simulink model "eps3"  (Simulink 8.3)
settings: Solver=ode3  SolverMode=SingleTasking  StartTime=0.0  StopTime=20  FixedStep=0.001  MaxStep=0.1  MinStep=0.01  RelTol=0.01
undefined symbols (not defined in the file or in its folder): Bc, Bm, G, Jc, Jm, Kc, Ke, Kt, L, R
libraries: fuzblock x2, Solver_SF x1
settings Model: Creator=xl  LastModifiedBy=汪天祥  CovMetricSettings=dwe  CovHtmlReporting=off  covSaveCumulativeToWorkspaceVar=off  CovSaveSingleToWorkspaceVar=off  CovExternalEMLEnable=on  CovSFcnEnable=on
settings SolverCC: InitialStep=0.01  ZeroCrossControl=EnableAll
settings DataIOCC: LimitDataPoints=off  SaveFormat=StructureWithTime  SignalLoggingSaveFormat=Dataset
settings DebuggingCC: UnderspecifiedInitializationDetection=Simplified  MergeDetectMultiDrivingBlocksExec=error  MaxConsecutiveZCsMsg=none  SolverPrmCheckMsg=none  FrameProcessingCompatibilityMsg=error  StateNameClashWarn=none  SFUnexpectedBacktrackingDiag=error  SFNoUnconditionalDefaultTransitionDiag=error
settings HardwareCC: ProdBitPerPointer=64  ProdLargestAtomicFloat=Float  ProdIntDivRoundTo=Zero  ProdEndianess=LittleEndian  ProdHWDeviceType=Specified
settings ModelReferenceCC: PropagateSignalLabelsOutOfModel=on
settings GRTTargetCC: TargetLangStandard=C99 (ISO)  GeneratePreprocessorConditionals=Use local settings  CombineOutputUpdateFcns=on  GRTInterface=off

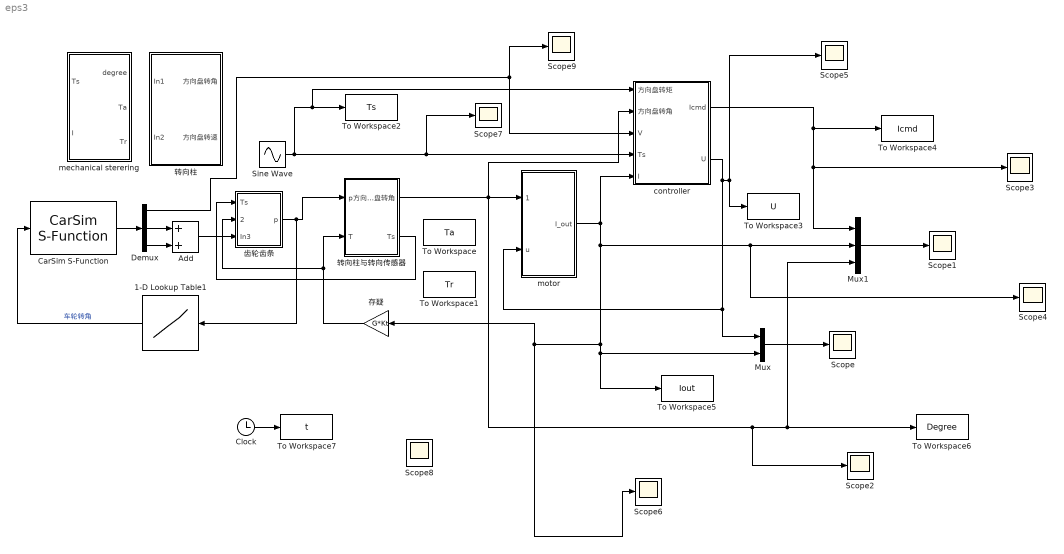
== system eps3 ==
  1-D Lookup Table1 : Lookup_n-D  NumberOfTableDimensions=1  BreakpointsForDimension1=[0 5 10 15 20 25 30 35 40 45 50 55 60 65 70 75 80]  Table=[2 4 6 8 10 12 14 16 18 20 22 24 27 29 31 33 36]  InternalRulePriority=Speed  RndMeth=Simplest  InputSameDT=on
  Add : Sum
  CarSim S-Function : Solver_SF/CarSim S-Function  Priority=1  VehicleCode=i_i  SIMFILE=simfile.sim
  Clock : Clock
  Demux : Demux  Outputs=3
  Mux : Mux  Inputs=2
  Mux1 : Mux  Inputs=3
  Scope{,1..9} (10 alike) : Scope
      Scope settings: YMin=-15.00000  YMax=15.00000
      Scope1 settings: YMin=-11.70772  YMax=11.82102
      Scope2 settings: YMin=-0.29342  YMax=0.29316
      Scope3 settings: YMin=-11.66423  YMax=11.66428  SaveName=ScopeData2  MaxDataPoints=10000
      Scope4 settings: YMin=-10  YMax=10  SaveName=ScopeData3
      Scope5 settings: YMin=-12.5  YMax=12.5  SaveName=ScopeData4
      Scope6 settings: YMin=-2.37496  YMax=2.36992  SaveName=ScopeData5
      Scope7 settings: YMin=-4.99999  YMax=5.00000  SaveName=ScopeData6
      Scope8 settings: YMin=-6.30329  YMax=6.29326  SaveName=ScopeData14
      Scope9 settings: YMin=-8.29353  YMax=8.28087  SaveName=ScopeData15
  Sine Wave : Sin  Amplitude=4  Frequency=1.333  SampleTime=0
  To Workspace : ToWorkspace  VariableName=Ta  SaveFormat=Timeseries  SampleTime=-1
  To Workspace1 : ToWorkspace  VariableName=Tr  SaveFormat=Timeseries  SampleTime=-1
  To Workspace2 : ToWorkspace  VariableName=Ts  SaveFormat=Timeseries  SampleTime=-1
  To Workspace3 : ToWorkspace  VariableName=U  SaveFormat=Timeseries  SampleTime=-1
  To Workspace4 : ToWorkspace  VariableName=Icmd  SaveFormat=Timeseries  SampleTime=-1
  To Workspace5 : ToWorkspace  VariableName=Iout  SaveFormat=Timeseries  SampleTime=-1
  To Workspace6 : ToWorkspace  VariableName=Degree  SaveFormat=Timeseries  SampleTime=-1
  To Workspace7 : ToWorkspace  VariableName=t  SaveFormat=Timeseries  SampleTime=-1
  "controller  " : Subsystem
  "mechanical sterering " : Subsystem
  "motor " : Subsystem
  存疑 : Gain  Gain=G*Kt
  转向柱 : Subsystem
  转向柱与转向传感器 : Subsystem
  齿轮齿条 : Subsystem
  wires:
  Sine Wave/1 -> "controller  "/1(方向盘转矩), To Workspace2/1, Scope7/1, "controller  "/4(Ts)
  "controller  "/2(U) -> "motor "/2(u), Mux/1, Scope5/1, To Workspace3/1
  "controller  "/1(Icmd) -> Scope3/1, Mux1/1, To Workspace4/1
  "motor "/1(I_out) -> Mux/2, To Workspace5/1, Scope6/1, 存疑/1, Scope4/1, Mux1/2, "controller  "/5(I)
  Mux/1 -> Scope/1
  Mux1/1 -> Scope1/1
  Clock/1 -> To Workspace7/1
  转向柱与转向传感器/1(方向盘转角) -> "controller  "/2(方向盘转角), "motor "/1("degree "), Scope2/1, To Workspace6/1, Mux1/3
  存疑/1 -> 转向柱与转向传感器/2(T), 齿轮齿条/2(电机转矩)
  齿轮齿条/1(p) -> 1-D Lookup Table1/1, 转向柱与转向传感器/1(p)
  转向柱与转向传感器/2(Ts) -> 齿轮齿条/1(Ts)
  Demux/1 -> Scope9/1, "controller  "/3(V)
  CarSim S-Function/1 -> Demux/1
  Demux/2 -> Add/1
  Demux/3 -> Add/2
  Add/1 -> 齿轮齿条/3(In3)
  1-D Lookup Table1/1 -> CarSim S-Function/1  "车轮转角"

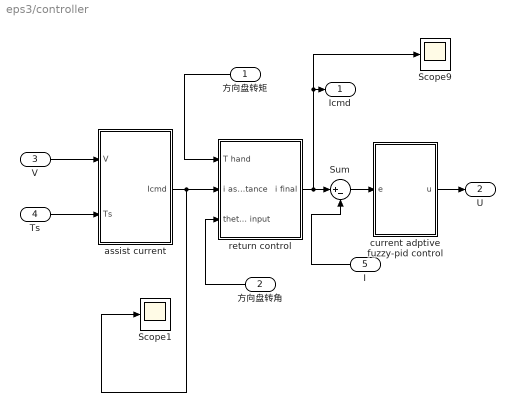
== system eps3/controller   ==
  方向盘转矩 : Inport
  方向盘转角 : Inport  Port=2
  V : Inport  Port=3
  Ts : Inport  Port=4
  I : Inport  Port=5
  Scope1 : Scope
      settings: YMin=-8.29353  YMax=8.28087  SaveName=ScopeData21
  Scope9 : Scope
      settings: YMin=-8.29353  YMax=8.28087  SaveName=ScopeData20
  Sum : Sum  Inputs=|+-
  "assist current " : Subsystem
  "current adptive fuzzy-pid control " : Subsystem
  "return control " : Subsystem
  Icmd : Outport
  U : Outport  Port=2
  wires:
  I/1 -> Sum/2
  "current adptive fuzzy-pid control "/1(u) -> U/1
  Sum/1 -> "current adptive fuzzy-pid control "/1("e ")
  V/1 -> "assist current "/1(V)
  Ts/1 -> "assist current "/2(Ts)
  方向盘转矩/1 -> "return control "/1("T hand ")
  方向盘转角/1 -> "return control "/3("theta input ")
  "assist current "/1(Icmd) -> Scope1/1, "return control "/2(i assitance)
  "return control "/1(i final) -> Scope9/1, Icmd/1, Sum/1

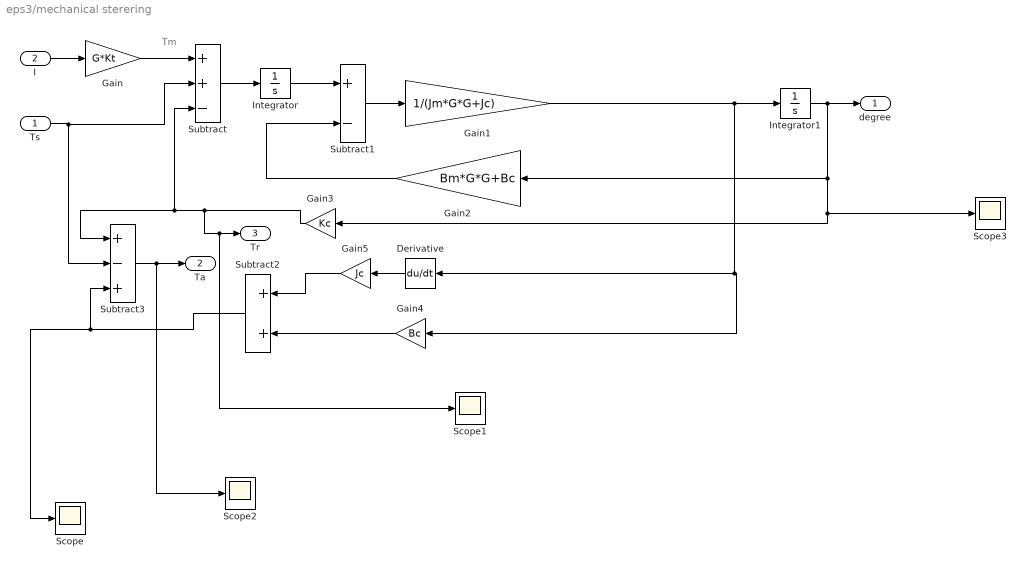
== system eps3/mechanical sterering  ==
  note: Tm
  Ts : Inport
  I : Inport  Port=2
  Derivative : Derivative
  Gain : Gain  Gain=G*Kt
  Gain1 : Gain  Gain=1/(Jm*G*G+Jc)
  Gain2 : Gain  Gain=Bm*G*G+Bc
  Gain3 : Gain  Gain=Kc
  Gain4 : Gain  Gain=Bc
  Gain5 : Gain  Gain=Jc
  Integrator : Integrator
  Integrator1 : Integrator
  Scope{,1..3} (4 alike) : Scope
      Scope settings: YMin=-0.17619  YMax=0.17432  SaveName=ScopeData16
      Scope1 settings: YMin=-13.24776  YMax=13.23609  SaveName=ScopeData17
      Scope2 settings: YMin=-8.29353  YMax=8.28087  SaveName=ScopeData18
      Scope3 settings: YMin=-0.13961  YMax=0.13939  SaveName=ScopeData19
  Subtract : Sum  Inputs=++-
  Subtract1 : Sum  Inputs=+-
  Subtract2 : Sum
  Subtract3 : Sum  Inputs=+-+
  "degree " : Outport
  Ta : Outport  Port=2
  Tr : Outport  Port=3
  wires:
  Subtract2/1 -> Scope/1, Subtract3/3
  Gain5/1 -> Subtract2/1
  Gain4/1 -> Subtract2/2
  Derivative/1 -> Gain5/1
  Gain2/1 -> Subtract1/2
  Integrator1/1 -> "degree "/1, Scope3/1, Gain3/1, Gain2/1
  Ts/1 -> Subtract/2, Subtract3/2
  Subtract3/1 -> Scope2/1, Ta/1
  Gain3/1 -> Scope1/1, Tr/1, Subtract3/1, Subtract/3
  Gain/1 -> Subtract/1
  Integrator/1 -> Subtract1/1
  Gain1/1 -> Derivative/1, Gain4/1, Integrator1/1
  I/1 -> Gain/1
  Subtract/1 -> Integrator/1
  Subtract1/1 -> Gain1/1

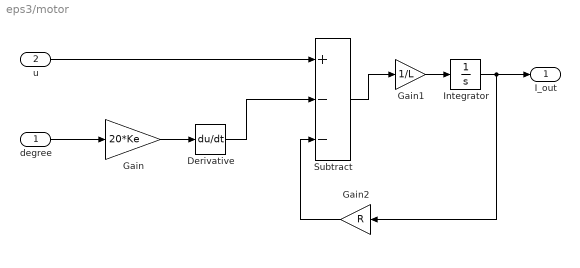
== system eps3/motor  ==
  "degree " : Inport
  u : Inport  Port=2
  Derivative : Derivative
  Gain : Gain  Gain=20*Ke
  Gain1 : Gain  Gain=1/L
  Gain2 : Gain  Gain=R
  Integrator : Integrator
  Subtract : Sum  Inputs=+--
  I_out : Outport
  wires:
  u/1 -> Subtract/1
  "degree "/1 -> Gain/1
  Derivative/1 -> Subtract/2
  Gain/1 -> Derivative/1
  Subtract/1 -> Gain1/1
  Gain2/1 -> Subtract/3
  Integrator/1 -> I_out/1, Gain2/1
  Gain1/1 -> Integrator/1

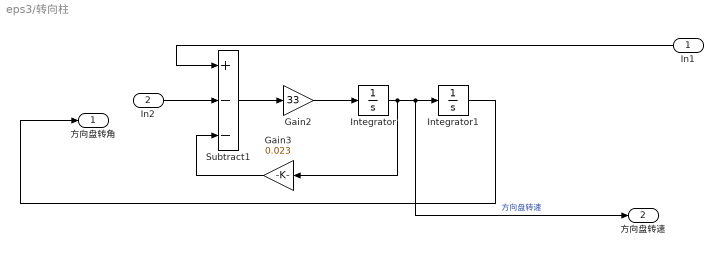
== system eps3/转向柱 ==
  In1 : Inport
  In2 : Inport  Port=2
  Gain2 : Gain  Gain=33
  Gain3 : Gain  Gain=0.023
  Integrator : Integrator
  Integrator1 : Integrator
  Subtract1 : Sum  Inputs=+--
  方向盘转角 : Outport
  方向盘转速 : Outport  Port=2
  wires:
  In2/1 -> Subtract1/2
  In1/1 -> Subtract1/1
  Integrator/1 -> Gain3/1, 方向盘转速/1, Integrator1/1  "方向盘转速"
  Integrator1/1 -> 方向盘转角/1
  Subtract1/1 -> Gain2/1
  Gain3/1 -> Subtract1/3
  Gain2/1 -> Integrator/1

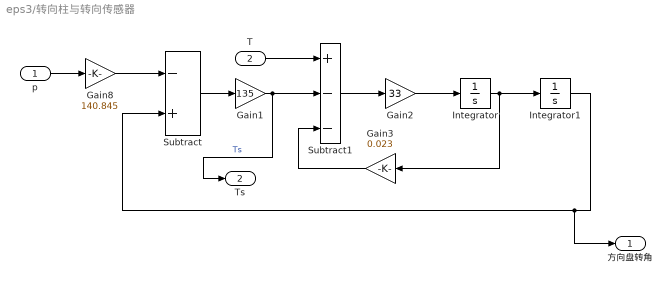
== system eps3/转向柱与转向传感器 ==
  p : Inport
  T : Inport  Port=2
  Gain1 : Gain  Gain=135
  Gain2 : Gain  Gain=33
  Gain3 : Gain  Gain=0.023
  Gain8 : Gain  Gain=140.845
  Integrator : Integrator
  Integrator1 : Integrator
  Subtract : Sum  Inputs=-+
  Subtract1 : Sum  Inputs=+--
  方向盘转角 : Outport
  Ts : Outport  Port=2
  wires:
  p/1 -> Gain8/1
  Gain1/1 -> Ts/1, Subtract1/2  "Ts"
  Gain2/1 -> Integrator/1
  Subtract/1 -> Gain1/1
  Subtract1/1 -> Gain2/1
  Integrator/1 -> Gain3/1, Integrator1/1
  T/1 -> Subtract1/1
  Integrator1/1 -> 方向盘转角/1, Subtract/2
  Gain3/1 -> Subtract1/3
  Gain8/1 -> Subtract/1

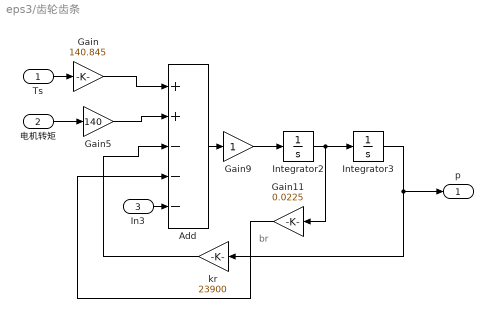
== system eps3/齿轮齿条 ==
  note: br
  Ts : Inport
  电机转矩 : Inport  Port=2
  In3 : Inport  Port=3
  Add : Sum  Inputs=++---
  Gain : Gain  Gain=140.845
  Gain11 : Gain  Gain=0.0225
  Gain5 : Gain  Gain=140
  Gain9 : Gain
  Integrator2 : Integrator
  Integrator3 : Integrator
  kr : Gain  Gain=23900
  p : Outport
  wires:
  Ts/1 -> Gain/1
  Add/1 -> Gain9/1
  Gain/1 -> Add/1
  kr/1 -> Add/3
  Gain5/1 -> Add/2
  Integrator2/1 -> Gain11/1, Integrator3/1
  Integrator3/1 -> p/1, kr/1
  Gain9/1 -> Integrator2/1
  Gain11/1 -> Add/4
  电机转矩/1 -> Gain5/1
  In3/1 -> Add/5

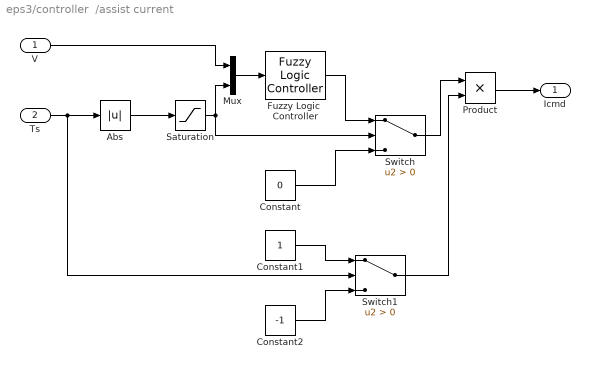
== system eps3/controller  /assist current  ==
  V : Inport
  Ts : Inport  Port=2
  Abs : Abs
  Constant : Constant  Value=0
  Constant1 : Constant
  Constant2 : Constant  Value=-1
  Fuzzy Logic  Controller : fuzblock/Fuzzy Logic  Controller  fis=assistcurrent
  Mux : Mux  Inputs=2
  Product : Product
  Saturation : Saturate  UpperLimit=80  LowerLimit=0
  Switch : Switch  Criteria=u2 > Threshold
  Switch1 : Switch  Criteria=u2 > Threshold
  Icmd : Outport
  wires:
  V/1 -> Mux/1
  Switch/1 -> Product/1
  Constant1/1 -> Switch1/1
  Switch1/1 -> Product/2
  Constant2/1 -> Switch1/3
  Mux/1 -> Fuzzy Logic  Controller/1
  Ts/1 -> Switch1/2, Abs/1
  Abs/1 -> Saturation/1
  Product/1 -> Icmd/1
  Saturation/1 -> Switch/2, Mux/2
  Constant/1 -> Switch/3
  Fuzzy Logic  Controller/1 -> Switch/1

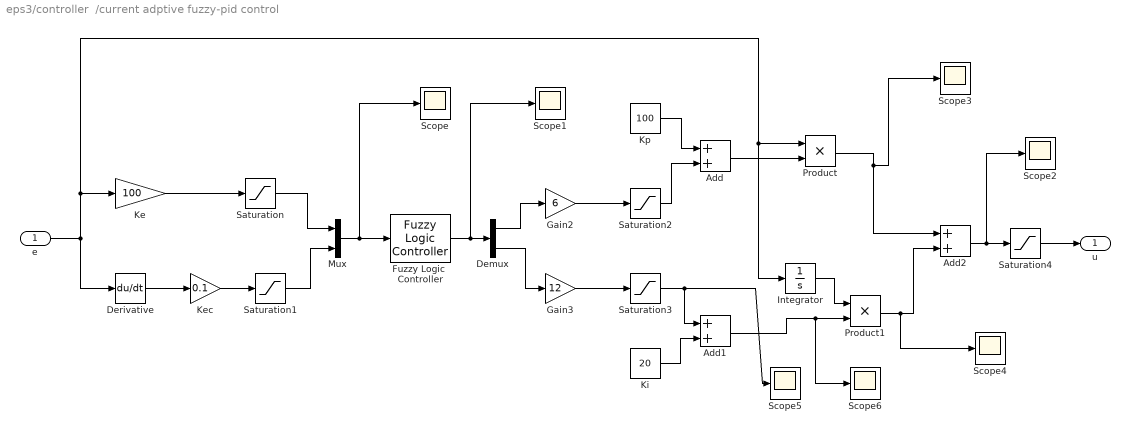
== system eps3/controller  /current adptive fuzzy-pid control  ==
  "e " : Inport
  Add : Sum
  Add1 : Sum
  Add2 : Sum
  Demux : Demux  Outputs=2
  Derivative : Derivative
  Fuzzy Logic  Controller : fuzblock/Fuzzy Logic  Controller  fis=adptivefuzzypidcontrol
  Gain2 : Gain  Gain=6
  Gain3 : Gain  Gain=12
  Integrator : Integrator
  Ke : Gain  Gain=100
  Kec : Gain  Gain=0.1
  Ki : Constant  Value=20
  Kp : Constant  Value=100
  Mux : Mux  Inputs=2
  Product : Product
  Product1 : Product
  Saturation{,1..3} (4 alike) : Saturate  UpperLimit=6  LowerLimit=-6
  Saturation4 : Saturate  UpperLimit=12  LowerLimit=-12
  Scope{,1..6} (7 alike) : Scope
      Scope settings: YMin=-7.5  YMax=7.5  SaveName=ScopeData7
      Scope1 settings: YMin=-6.71538  YMax=6.71538  SaveName=ScopeData8
      Scope2 settings: YMin=-80.22694  YMax=672.92649  SaveName=ScopeData9
      Scope3 settings: YMin=-80.64056  YMax=672.97051  SaveName=ScopeData10
      Scope4 settings: YMin=-80.64056  YMax=672.97051  SaveName=ScopeData11
      Scope5 settings: YMin=-80.64056  YMax=672.97051  SaveName=ScopeData12
      Scope6 settings: YMin=2.5  YMax=17.5  SaveName=ScopeData13
  u : Outport
  wires:
  Kec/1 -> Saturation1/1
  Derivative/1 -> Kec/1
  Gain3/1 -> Saturation3/1
  Ki/1 -> Add1/2
  Saturation4/1 -> u/1
  "e "/1 -> Derivative/1, Product/1, Integrator/1, Ke/1
  Mux/1 -> Scope/1, Fuzzy Logic  Controller/1
  Saturation3/1 -> Scope5/1, Add1/1
  Add/1 -> Product/2
  Fuzzy Logic  Controller/1 -> Scope1/1, Demux/1
  Demux/2 -> Gain3/1
  Product/1 -> Scope3/1, Add2/1
  Product1/1 -> Scope4/1, Add2/2
  Add2/1 -> Scope2/1, Saturation4/1
  Saturation/1 -> Mux/1
  Saturation1/1 -> Mux/2
  Integrator/1 -> Product1/1
  Add1/1 -> Scope6/1, Product1/2
  Gain2/1 -> Saturation2/1
  Demux/1 -> Gain2/1
  Saturation2/1 -> Add/2
  Kp/1 -> Add/1
  Ke/1 -> Saturation/1

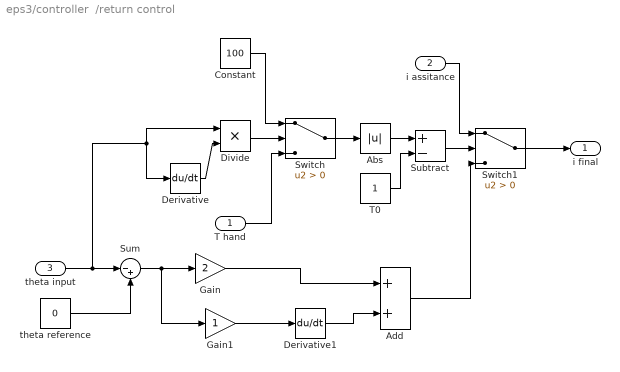
== system eps3/controller  /return control  ==
  "T hand " : Inport
  i assitance : Inport  Port=2
  "theta input " : Inport  Port=3
  Abs : Abs
  Add : Sum
  Constant : Constant  Value=100
  Derivative : Derivative
  Derivative1 : Derivative
  Divide : Product  Inputs=**
  Gain : Gain  Gain=2
  Gain1 : Gain
  Subtract : Sum  Inputs=+-
  Sum : Sum  Inputs=|-+
  Switch : Switch  Criteria=u2 > Threshold
  Switch1 : Switch  Criteria=u2 > Threshold
  "T0 " : Constant
  theta reference : Constant  Value=0
  i final : Outport
  wires:
  "T hand "/1 -> Switch/3
  "theta input "/1 -> Sum/1, Divide/1, Derivative/1
  Sum/1 -> Gain/1, Gain1/1
  Gain1/1 -> Derivative1/1
  Switch1/1 -> i final/1
  theta reference/1 -> Sum/2
  Derivative1/1 -> Add/2
  Add/1 -> Switch1/3
  Gain/1 -> Add/1
  i assitance/1 -> Switch1/1
  Subtract/1 -> Switch1/2
  "T0 "/1 -> Subtract/2
  Abs/1 -> Subtract/1
  Constant/1 -> Switch/1
  Divide/1 -> Switch/2
  Derivative/1 -> Divide/2
  Switch/1 -> Abs/1
